simulink model "sampleModel1820"  (R2023a)
settings: Solver=VariableStepAuto  StartTime=0.0  StopTime=10.0  RelTol=1e-3
libraries: hdlsllib x5, simulink x2
settings Model: Creator=user1  LastModifiedBy=user1

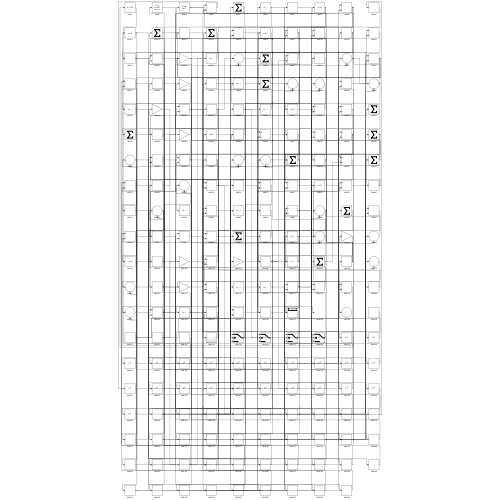
[thumbnail: Simulink's stored preview of the top-level diagram]
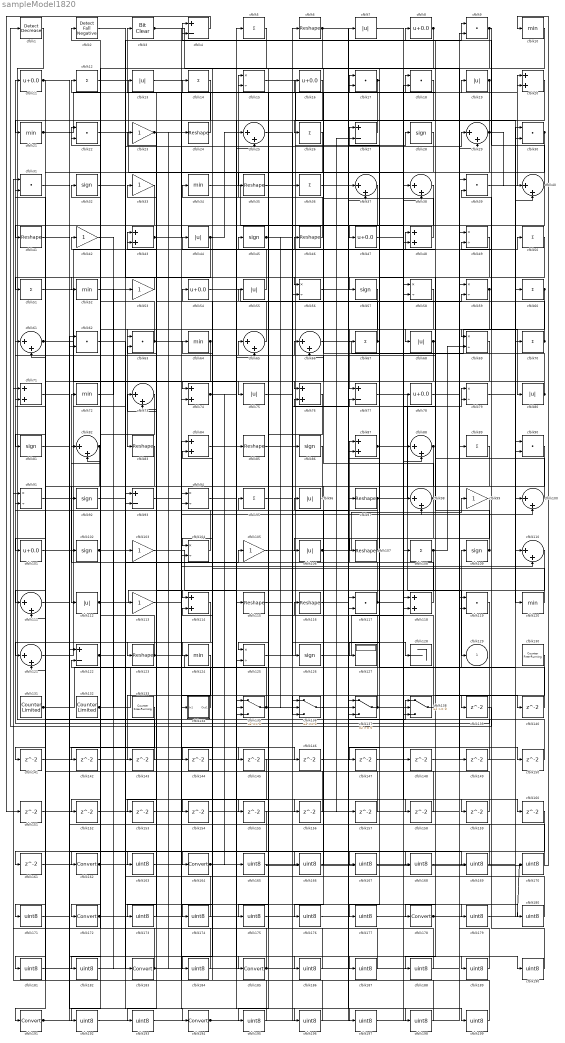
== system sampleModel1820 ==
  cfblk1 : simulink/Logic and Bit Operations/Detect Decrease  vinit=0.0  OutDataTypeStr=boolean
      settings: LibrarySourceBlock=|
      | hdlsllib/Logic and Bit
      | Operations/Detect
      | Decrease
  cfblk{10,21,34,52,64,72,120,124} (8 alike) : MinMax
  cfblk{25,29,37..38,40,61,65..66,73,82,88,98,100,110..111,121} (16 alike) : Sum  Inputs=|++
  cfblk{8,11,16,47,54,78,101} (7 alike) : Bias  Bias=0.0  SaturateOnIntegerOverflow=off
  cfblk{28,32,45,57,81,86,92,102,109,126} (10 alike) : Signum
  cfblk{23,33,42,53,99,103,105,113} (8 alike) : Gain
  cfblk{15,49,56,58..59,69,79,91,94,104,125} (11 alike) : Product  Inputs=*/  RndMeth=Zero  SaturateOnIntegerOverflow=on
  cfblk{7,13,19,44,55,68,75,80,96,106,112} (11 alike) : Abs  SaturateOnIntegerOverflow=off
  cfblk{6,24,35,41,46,83,85,97,107,115..116,123} (12 alike) : Reshape
  cfblk{5,12,14,26,36,50..51,60,67,70,89,95,108} (13 alike) : Sum  Inputs=+
  cfblk{20,43,48,71,74,76,84,87,114,118} (10 alike) : Sum
  cfblk{9,17..18,22,30..31,39,62..63,90,117,119} (12 alike) : DotProduct  OutDataTypeStr=Inherit: Inherit via internal rule
  cfblk{4,27,77,93,122} (5 alike) : Sum  Inputs=+-
  cfblk127 : Display
  cfblk128 : Terminator
  cfblk130 : hdlsllib/Sources/Counter Free-Running  NumBits=16  tsamp=-1
  cfblk131 : hdlsllib/Sources/Counter Limited  uplimit=7  tsamp=-1
  cfblk132 : hdlsllib/Sources/Counter Limited  uplimit=7  tsamp=-1
  cfblk133 : hdlsllib/Sources/Counter Free-Running  NumBits=16  tsamp=-1
  cfblk134 : Subsystem
      settings: LibrarySourceBlock=|
      | hdlsllib/Ports &
      | Subsystems/Subsystem
  cfblk{135..138} (4 alike) : Switch  SaturateOnIntegerOverflow=off  InputSameDT=off
  cfblk{139..161} (23 alike) : Delay  SampleTime=1
  cfblk{162,164,172,178,183,185,191,194} (8 alike) : DataTypeConversion  SaturateOnIntegerOverflow=off  RndMeth=Floor
  cfblk{163,165..171,173..177,179..182,184,186..190,192..193,195..199} (30 alike) : DataTypeConversion  OutDataTypeStr=uint8  SaturateOnIntegerOverflow=off  RndMeth=Floor
  cfblk2 : hdlsllib/Logic and Bit Operations/Detect Fall Negative  vinit=0  OutDataTypeStr=boolean
  cfblk3 : simulink/Logic and Bit Operations/Bit Clear  iBit=0
      settings: LibrarySourceBlock=|
      | hdlsllib/Logic and Bit
      | Operations/Bit Clear
  cfblk129 : Outport  VectorParamsAs1DForOutWhenUnconnected=off
  wires:
  cfblk125/1 -> cfblk48/1
  cfblk68/1 -> cfblk14/1, cfblk135/2
  cfblk66/1 -> cfblk80/1
  cfblk55/1 -> cfblk45/1
  cfblk132/1 -> cfblk103/1, cfblk115/1
  cfblk112/1 -> cfblk114/1, cfblk199/1
  cfblk123/1 -> cfblk109/1, cfblk138/3, cfblk22/1, cfblk163/1
  cfblk8/1 -> cfblk118/2, cfblk66/2
  cfblk97/1 -> cfblk79/1, cfblk91/2
  cfblk77/1 -> cfblk129/1
  cfblk34/1 -> cfblk48/2
  cfblk6/1 -> cfblk75/1, cfblk58/2
  cfblk10/1 -> cfblk164/1
  cfblk1/1 -> cfblk138/1
  cfblk85/1 -> cfblk19/1
  cfblk72/1 -> cfblk53/1
  cfblk79/1 -> cfblk110/1
  cfblk119/1 -> cfblk11/1
  cfblk61/1 -> cfblk125/2, cfblk181/1
  cfblk73/1 -> cfblk172/1
  cfblk24/1 -> cfblk3/1
  cfblk109/1 -> cfblk44/1, cfblk76/2, cfblk4/2
  cfblk65/1 -> cfblk33/1
  cfblk40/1 -> cfblk125/1, cfblk4/1
  cfblk54/1 -> cfblk59/2
  cfblk16/1 -> cfblk104/1
  cfblk52/1 -> cfblk9/1
  cfblk59/1 -> cfblk83/1, cfblk82/2
  cfblk60/1 -> cfblk77/1, cfblk68/1
  cfblk88/1 -> cfblk124/1, cfblk144/1
  cfblk91/1 -> cfblk43/1
  cfblk27/1 -> cfblk26/1
  cfblk5/1 -> cfblk162/1
  cfblk117/1 -> cfblk72/1, cfblk88/2, cfblk79/2
  cfblk32/1 -> cfblk57/1
  cfblk12/1 -> cfblk98/1
  cfblk131/1 -> cfblk70/1, cfblk113/1
  cfblk43/1 -> cfblk110/2, cfblk17/1
  cfblk39/1 -> cfblk20/1
  cfblk134/1(Out1) -> cfblk32/1
  cfblk63/1 -> cfblk12/1, cfblk136/3
  cfblk130/1 -> cfblk178/1
  cfblk15/1 -> cfblk120/1
  cfblk102/1 -> cfblk46/1, cfblk22/2
  cfblk120/1 -> cfblk64/1
  cfblk23/1 -> cfblk145/1, cfblk193/1
  cfblk28/1 -> cfblk123/1
  cfblk33/1 -> cfblk81/1
  cfblk118/1 -> cfblk87/1
  cfblk35/1 -> cfblk28/1
  cfblk20/1 -> cfblk119/2
  cfblk121/1 -> cfblk29/1
  cfblk31/1 -> cfblk185/1
  cfblk51/1 -> cfblk134/1(In1)
  cfblk14/1 -> cfblk41/1
  cfblk137/1 -> cfblk65/1, cfblk140/1
  cfblk22/1 -> cfblk94/1
  cfblk3/1 -> cfblk89/1, cfblk158/1
  cfblk46/1 -> cfblk15/1
  cfblk98/1 -> cfblk66/1, cfblk147/1
  cfblk53/1 -> cfblk51/1
  cfblk101/1 -> cfblk8/1
  cfblk75/1 -> cfblk126/1
  cfblk138/1 -> cfblk96/1
  cfblk71/1 -> cfblk194/1
  cfblk106/1 -> cfblk99/1, cfblk27/2, cfblk157/1
  cfblk26/1 -> cfblk35/1
  cfblk108/1 -> cfblk137/3, cfblk69/2
  cfblk107/1 -> cfblk27/1, cfblk95/1
  cfblk45/1 -> cfblk6/1, cfblk136/2
  cfblk135/1 -> cfblk36/1, cfblk63/2
  cfblk17/1 -> cfblk47/1, cfblk76/1
  cfblk56/1 -> cfblk100/2
  cfblk105/1 -> cfblk97/1
  cfblk48/1 -> cfblk16/1
  cfblk82/1 -> cfblk112/1, cfblk161/1
  cfblk70/1 -> cfblk18/1, cfblk15/2
  cfblk115/1 -> cfblk20/2
  cfblk7/1 -> cfblk88/1
  cfblk9/1 -> cfblk69/1, cfblk117/2, cfblk177/1
  cfblk25/1 -> cfblk128/1
  cfblk104/1 -> cfblk13/1
  cfblk89/1 -> cfblk106/1
  cfblk50/1 -> cfblk67/1
  cfblk122/1 -> cfblk105/1, cfblk160/1
  cfblk64/1 -> cfblk111/1, cfblk104/2
  cfblk37/1 -> cfblk191/1
  cfblk11/1 -> cfblk101/1, cfblk168/1
  cfblk113/1 -> cfblk98/2
  cfblk74/1 -> cfblk138/2, cfblk165/1
  cfblk21/1 -> cfblk17/2, cfblk190/1
  cfblk114/1 -> cfblk121/1
  cfblk103/1 -> cfblk135/1
  cfblk41/1 -> cfblk102/1
  cfblk80/1 -> cfblk74/1, cfblk34/1
  cfblk44/1 -> cfblk52/1, cfblk25/1, cfblk154/1
  cfblk42/1 -> cfblk183/1
  cfblk96/1 -> cfblk92/1
  cfblk95/1 -> cfblk77/2
  cfblk29/1 -> cfblk21/1, cfblk40/1, cfblk94/2
  cfblk87/1 -> cfblk108/1, cfblk50/1
  cfblk100/1 -> cfblk61/1
  cfblk67/1 -> cfblk107/1, cfblk43/2
  cfblk2/1 -> cfblk56/1
  cfblk19/1 -> cfblk74/2, cfblk135/3
  cfblk126/1 -> cfblk18/2
  cfblk30/1 -> cfblk111/2, cfblk63/1, cfblk127/1
  cfblk116/1 -> cfblk139/1
  cfblk139/1 -> cfblk1/1
  cfblk140/1 -> cfblk87/2
  cfblk83/1 -> cfblk141/1
  cfblk141/1 -> cfblk118/1
  cfblk18/1 -> cfblk142/1
  cfblk142/1 -> cfblk29/2
  cfblk124/1 -> cfblk143/1
  cfblk143/1 -> cfblk121/2
  cfblk144/1 -> cfblk114/2
  cfblk111/1 -> cfblk146/1
  cfblk147/1 -> cfblk100/1
  cfblk148/1 -> cfblk119/1
  cfblk78/1 -> cfblk149/1
  cfblk149/1 -> cfblk137/2
  cfblk136/1 -> cfblk150/1
  cfblk150/1 -> cfblk137/1
  cfblk4/1 -> cfblk151/1
  cfblk151/1 -> cfblk59/1
  cfblk69/1 -> cfblk152/1
  cfblk110/1 -> cfblk153/1
  cfblk154/1 -> cfblk56/2
  cfblk76/1 -> cfblk155/1
  cfblk94/1 -> cfblk156/1
  cfblk156/1 -> cfblk82/1
  cfblk157/1 -> cfblk61/2
  cfblk158/1 -> cfblk58/1
  cfblk47/1 -> cfblk159/1
  cfblk159/1 -> cfblk2/1
  cfblk161/1 -> cfblk65/2
  cfblk162/1 -> cfblk85/1, cfblk117/1
  cfblk163/1 -> cfblk5/1
  cfblk164/1 -> cfblk148/1, cfblk40/2
  cfblk165/1 -> cfblk10/1
  cfblk90/1 -> cfblk166/1
  cfblk166/1 -> cfblk116/1
  cfblk92/1 -> cfblk167/1
  cfblk167/1 -> cfblk90/1
  cfblk168/1 -> cfblk90/2
  cfblk62/1 -> cfblk169/1
  cfblk169/1 -> cfblk23/1
  cfblk170/1 -> cfblk62/1
  cfblk160/1 -> cfblk171/1
  cfblk171/1 -> cfblk62/2
  cfblk172/1 -> cfblk170/1, cfblk7/1
  cfblk58/1 -> cfblk173/1
  cfblk173/1 -> cfblk73/1
  cfblk145/1 -> cfblk174/1
  cfblk174/1 -> cfblk73/2
  cfblk38/1 -> cfblk175/1
  cfblk175/1 -> cfblk30/2
  cfblk99/1 -> cfblk176/1
  cfblk176/1 -> cfblk38/1
  cfblk177/1 -> cfblk38/2
  cfblk178/1 -> cfblk60/1, cfblk30/1
  cfblk93/1 -> cfblk179/1
  cfblk179/1 -> cfblk39/2
  cfblk152/1 -> cfblk180/1
  cfblk180/1 -> cfblk93/1
  cfblk181/1 -> cfblk93/2
  cfblk133/1 -> cfblk182/1
  cfblk182/1 -> cfblk39/1
  cfblk183/1 -> cfblk25/2, cfblk122/2, cfblk24/1
  cfblk86/1 -> cfblk184/1
  cfblk184/1 -> cfblk42/1
  cfblk185/1 -> cfblk91/1, cfblk54/1
  cfblk81/1 -> cfblk186/1
  cfblk186/1 -> cfblk31/1
  cfblk153/1 -> cfblk187/1
  cfblk187/1 -> cfblk31/2
  cfblk49/1 -> cfblk188/1
  cfblk188/1 -> cfblk55/1
  cfblk146/1 -> cfblk189/1
  cfblk189/1 -> cfblk49/1
  cfblk190/1 -> cfblk49/2
  cfblk191/1 -> cfblk122/1, cfblk86/1
  cfblk155/1 -> cfblk192/1
  cfblk192/1 -> cfblk37/1
  cfblk193/1 -> cfblk37/2
  cfblk194/1 -> cfblk136/1, cfblk78/1
  cfblk57/1 -> cfblk195/1
  cfblk195/1 -> cfblk71/1
  cfblk13/1 -> cfblk196/1
  cfblk196/1 -> cfblk71/2
  cfblk84/1 -> cfblk197/1
  cfblk197/1 -> cfblk9/2
  cfblk36/1 -> cfblk198/1
  cfblk198/1 -> cfblk84/1
  cfblk199/1 -> cfblk84/2

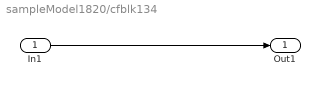
== system sampleModel1820/cfblk134 ==
  In1 : Inport
  Out1 : Outport
  wires:
  In1/1 -> Out1/1
